simulink library "Ground_Source_Heat_Exchanger"  (R2018b)
settings: Solver=ode45  StartTime=0.0  StopTime=10.0  RelTol=1e-3  EnableMultiTasking=on
undefined symbols (not defined in the file): Ad, Ad0, Ar, Au, Au0, Bd, Bd0, Br, Bu, Bu0, c1, c33, c4, Cd, Cdl, Cr, Cu, Dd, DiameterLastPiece, dl, Dr, Du, gfunction, L1, r_Trichter, Rechenradius, T_null, t_start, t_Trichter, Tdown_0, Tearth_anf, Temperature, Tup_0
settings Model: Creator=lena.frank  LastModifiedBy=drhf
settings DataIOCC: LimitDataPoints=on  SaveFormat=Array  SignalLoggingSaveFormat=ModelDataLogs
settings OptimizationCC: ExpressionDepthLimit=2147483647  LifeSpan=inf
settings DebuggingCC: UnderspecifiedInitializationDetection=Classic  MergeDetectMultiDrivingBlocksExec=none  SolverPrmCheckMsg=warning  FcnCallInpInsideContextMsg=warning  StateNameClashWarn=warning  SFUnexpectedBacktrackingDiag=warning  SFNoUnconditionalDefaultTransitionDiag=warning  SFExecutionAtInitializationDiag=none
settings HardwareCC: ProdBitPerPointer=32  ProdBitPerSizeT=32  ProdBitPerPtrDiffT=32  ProdLargestAtomicFloat=None  ProdIntDivRoundTo=Undefined  ProdEndianess=Unspecified  ProdWordSize=32  ProdHWDeviceType=32-bit Generic
settings ModelReferenceCC: PropagateSignalLabelsOutOfModel=off
settings SFSimCC: SimUseLocalCustomCode=off
settings RTWCC: RTWUseLocalCustomCode=off
settings CodeAppCC: StateflowObjectComments=on
settings GRTTargetCC: TargetLangStandard=C89/C90 (ANSI)  GeneratePreprocessorConditionals=Disable all  CombineOutputUpdateFcns=off  GRTInterface=on
settings ConfigComp: CovMetricSettings=dw  CovHtmlReporting=on  CovSaveCumulativeToWorkspaceVar=on  CovSaveSingleToWorkspaceVar=on  CovExternalEMLEnable=off

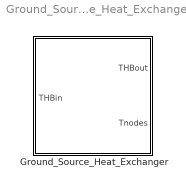
== system Ground_Source_Heat_Exchanger ==
  Ground_Source_Heat_Exchanger : Subsystem  mask(ground source heat exchanger){Jahresmitteltemp_C=10, TGrad=0.025, lambdaErde=2.5, cpErde=1000, rhoErde=2200, lambdaFill=0.81, cpFill=3040, rhoFill=1180, lambda_Sondenrohr=0.48, dTdesign=5, Sondenlaenge=100, B_sondenabstand=10, Sondendurchmesser=0.026+2*0.003, Bohrdurchmesser=0.12, Bu_param=0.06, Wanddicke_Sondenrohr=0.003, SondenFall=5x10 probes B/H = 0.1, DimVert=5, DimRad=10, Gitterfaktor=2.5, LastYear=1, show=off}
      mask prompts: Jahresmitteltemp_C "Average annual outdoor temperature  in °C"; TGrad "Temperature gradient in K/m, typical 0.025..0.04"; lambdaErde "Thermal conductivity ground in W/m/K"; cpErde "Heat capacity of the ground in J/kg/K"; rhoErde "Denstiy of the ground in kg/m³"; lambdaFill "Thermal conductivity filling in W/m/K"; cpFill "Heat capacity of the filling in J/kg/K"; rhoFill "Denstiy of the filling in kg/m³"; lambda_Sondenrohr "Thermal conductivity of pipe material  in W/m/K"; dTdesign "Design temperature difference inlet-outlet in K"; Sondenlaenge "H: Length of earth probe in m"; B_sondenabstand "B: Probe distance in m (= calculation diameter for single probe)"; Sondendurchmesser "Diameter of tube in m"; Bohrdurchmesser "Diameter of drilled hole in m"; Bu_param "Shank spacing in m (must be < borehole diameter)"; Wanddicke_Sondenrohr "Thickness of pipe wall in m"; SondenFall "Field geometry"; DimVert "No. of vertical nodes (typical 5, minimum 2)"; DimRad "No. of horizontal (radial) nodes (typical 10, minimum 3)"; Gitterfaktor "grid factor (typical 2.5, must be > 1)"; LastYear "Year of ground temperature pre-calculation (steady state = 50)"; show "Display start conditions"
      mask help: The CARNOT EWS model is a transient model for dynamic simulation of borehole heat exchangers or so-called vertical ground heat exchangers. The model is based on the equations described by [Huber] and has been implemented using the state space model of Matlab/Simulink [Bianchi]. See <Help> for literature.
      mask init:
      | startfall = 2;
      | DimAxi = max(DimVert*2,4);
      | DimRad = max(DimRad,3);
      | 
      | [Ad,Bd,Cd,Dd, Au,Bu,Cu,Du, Ad0,Bd0, Au0,Bu0, ...
      |     Ar,Br,Cr,Dr, Cdl, c1, c3, c31, c33, c4, c41, c5, c6, ...
      |     L1, L2, L10, L20, dl, Rechenradius, np, ...
      |     Tearth_anf, T_null, teta_fluid_ini, Tdown_0, Tup_0, ...
      |     Ts_Trichter, t_Trichter, r_Trichter, gfunction, t_start ...
      |     ] = ...
      |     CarnotCallbacks_EWS(startfall, LastYear, dTdesign, ...
      |     SondenFall, B_sondenabstand, Sondenlaenge, Sondendurchmesser, ...
      |     Bohrdurchmesser, Bu_param, Wanddicke_Sondenrohr, ...
      |     Jahresmitteltemp_C, TGrad, ...
      |     lambdaErde, rhoErde, cpErde, ...
      |     lambdaFill, cpFill, rhoFill, lambda_Sondenrohr, ...
      |     DimAxi, DimRad, Gitterfaktor, show);
      mask Help: web(fullfile(path_carnot('help'),'Ground_Source_Heat_Exchanger.html'),'-helpbrowser')
      mask TypeOptions SondenFall: 1 probe | 2 probes B/H = 0.1 | 2 probes B/H = 0.05 | 3x6 probes B/H = 0.1 | 5x10 probes B/H = 0.1
      mask DialogControl ParameterTabVar0 Prompt: Thermal
      mask DialogControl ParameterTabVar01 Prompt: Geometry
      mask DialogControl ParameterTabVar012 Prompt: Calculation
      mask Display:
      | plot(0,10,100,90,[70,30],[80,80], ...
      |     [35,35,43,43,47,52,57,57,66,66,60,60,54,46,40,40,35], ...
      |     [84,87,87,20,13,13,21,87,87,84,84,20,10,10,20,84,84])

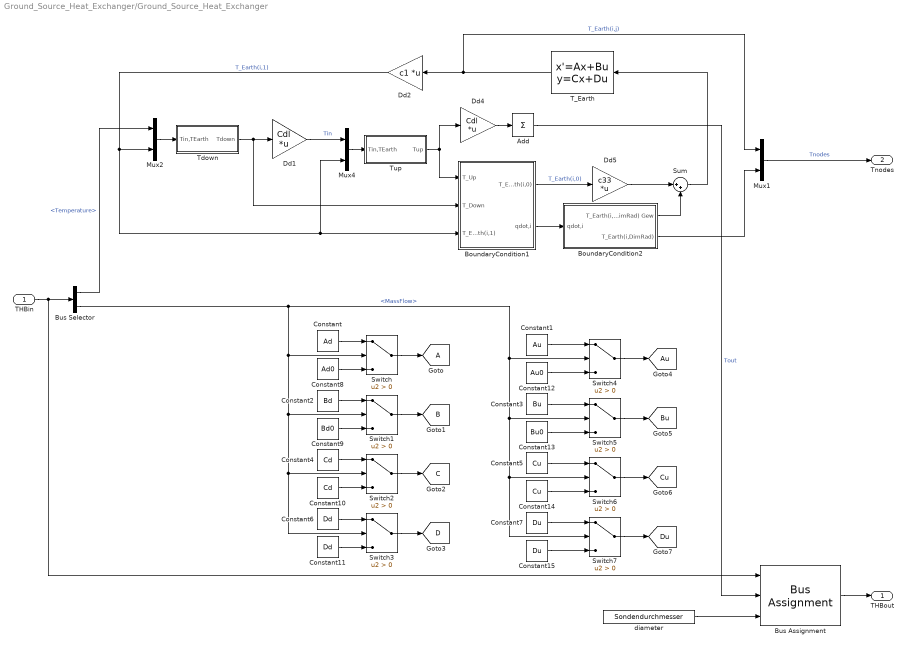
== system Ground_Source_Heat_Exchanger/Ground_Source_Heat_Exchanger ==
  THBin : Inport
  Add : Sum  Inputs=1
  BoundaryCondition1 : Subsystem
  BoundaryCondition2 : Subsystem
  Bus Assignment : BusAssignment  AssignedSignals=Temperature,DiameterLastPiece
  Bus Selector : BusSelector  OutputSignals=Temperature,MassFlow
  Constant : Constant  Value=Ad
  Constant1 : Constant  Value=Au
  Constant10 : Constant  Value=Cd
  Constant11 : Constant  Value=Dd
  Constant12 : Constant  Value=Au0
  Constant13 : Constant  Value=Bu0
  Constant14 : Constant  Value=Cu
  Constant15 : Constant  Value=Du
  Constant2 : Constant  Value=Bd
  Constant3 : Constant  Value=Bu
  Constant4 : Constant  Value=Cd
  Constant5 : Constant  Value=Cu
  Constant6 : Constant  Value=Dd
  Constant7 : Constant  Value=Du
  Constant8 : Constant  Value=Ad0
  Constant9 : Constant  Value=Bd0
  Dd1 : Gain  Gain=Cdl  Multiplication=Matrix(K*u)  SaturateOnIntegerOverflow=on  OutDataTypeStr=Inherit: Same as input  ParamDataTypeStr=Inherit: Same as input
  Dd2 : Gain  Gain=c1  Multiplication=Matrix(K*u)  SaturateOnIntegerOverflow=on  OutDataTypeStr=Inherit: Same as input  ParamDataTypeStr=Inherit: Same as input
  Dd4 : Gain  Gain=Cdl  Multiplication=Matrix(K*u)  SaturateOnIntegerOverflow=on  OutDataTypeStr=Inherit: Same as input  ParamDataTypeStr=Inherit: Same as input
  Dd5 : Gain  Gain=c33  Multiplication=Matrix(K*u)  SaturateOnIntegerOverflow=on  OutDataTypeStr=Inherit: Same as input  ParamDataTypeStr=Inherit: Same as input
  Mux1 : Mux  Inputs=2
  Mux2 : Mux  Inputs=2
  Mux4 : Mux  Inputs=2
  Sum : Sum  Inputs=|++  SaturateOnIntegerOverflow=on  InputSameDT=on  OutDataTypeStr=Inherit: Same as first input
  Switch{,1..7} (8 alike) : Switch  Criteria=u2 > Threshold
  T_Earth : StateSpace  A=Ar  B=Br  C=Cr  D=Dr  InitialCondition=Tearth_anf(:)
  Tdown : Subsystem
  Tup : Subsystem
  diameter : Constant  Value=Sondendurchmesser
  THBout : Outport
  Tnodes : Outport  Port=2
  tag scope: A=global, Au=global, B=global, Bu=global, C=global, Cu=global, D=global, Du=global
  wires:
  Bus Selector/1 -> Mux2/1  "<Temperature>"
  Bus Selector/2 -> Switch4/2, Switch5/2, Switch7/2, Switch6/2, Switch/2, Switch1/2, Switch3/2, Switch2/2  "<MassFlow>"
  Constant12/1 -> Switch4/3
  Constant13/1 -> Switch5/3
  Constant14/1 -> Switch6/3
  Constant15/1 -> Switch7/3
  Switch4/1 -> [Au]
  Switch5/1 -> [Bu]
  Switch6/1 -> [Cu]
  Switch7/1 -> [Du]
  Constant7/1 -> Switch7/1
  Constant5/1 -> Switch6/1
  Constant3/1 -> Switch5/1
  Constant1/1 -> Switch4/1
  Constant6/1 -> Switch3/1
  Constant11/1 -> Switch3/3
  Constant10/1 -> Switch2/3
  Switch3/1 -> [D]
  Constant4/1 -> Switch2/1
  Switch2/1 -> [C]
  Constant9/1 -> Switch1/3
  Constant2/1 -> Switch1/1
  Constant/1 -> Switch/1
  Switch1/1 -> [B]
  Constant8/1 -> Switch/3
  Switch/1 -> [A]
  Tdown/1(Tdown) -> Dd1/1, BoundaryCondition1/2(T_Down)
  Mux2/1 -> Tdown/1(Tin,TEarth)
  Mux4/1 -> Tup/1(Tin,TEarth)
  Dd1/1 -> Mux4/1  "Tin"
  T_Earth/1 -> Dd2/1, Mux1/1  "T_Earth(i,j)"
  Tup/1(Tup) -> Dd4/1, BoundaryCondition1/1(T_Up)
  Dd5/1 -> Sum/1
  BoundaryCondition2/1(T_Earth(i,DimRad) Gew) -> Sum/2
  Sum/1 -> T_Earth/1
  BoundaryCondition1/1(T_Earth(i,0)) -> Dd5/1  "T_Earth(i,0)"
  Dd2/1 -> Mux4/2, BoundaryCondition1/3(T_Earth(i,1)), Mux2/2  "T_Earth(i,1)"
  BoundaryCondition2/2(T_Earth(i,DimRad)) -> Mux1/2
  THBin/1 -> Bus Selector/1, Bus Assignment/1
  diameter/1 -> Bus Assignment/3
  Bus Assignment/1 -> THBout/1
  Dd4/1 -> Add/1
  Add/1 -> Bus Assignment/2  "Tout"
  Mux1/1 -> Tnodes/1  "Tnodes"
  BoundaryCondition1/2(qdot,i) -> BoundaryCondition2/1(qdot,i)

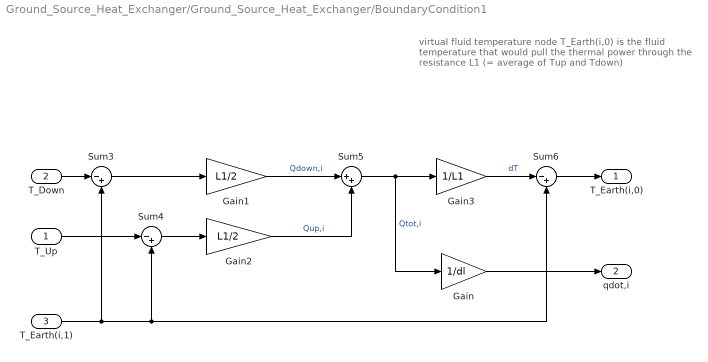
== system Ground_Source_Heat_Exchanger/Ground_Source_Heat_Exchanger/BoundaryCondition1 ==
  note: virtual fluid temperature node T_Earth(i,0) is the
      | fluid temperature that would pull the thermal
      | power through the resistance L1 (= average of
      | Tup and Tdown)
  T_Up : Inport
  T_Down : Inport  Port=2
  T_Earth(i,1) : Inport  Port=3
  Gain : Gain  Gain=1/dl
  Gain1 : Gain  Gain=L1/2  SaturateOnIntegerOverflow=on  OutDataTypeStr=Inherit: Same as input  ParamDataTypeStr=Inherit: Same as input
  Gain2 : Gain  Gain=L1/2  SaturateOnIntegerOverflow=on  OutDataTypeStr=Inherit: Same as input  ParamDataTypeStr=Inherit: Same as input
  Gain3 : Gain  Gain=1/L1  SaturateOnIntegerOverflow=on  OutDataTypeStr=Inherit: Same as input  ParamDataTypeStr=Inherit: Same as input
  Sum3 : Sum  Inputs=|-+  SaturateOnIntegerOverflow=on  InputSameDT=on  OutDataTypeStr=Inherit: Same as first input
  Sum4 : Sum  Inputs=|-+  SaturateOnIntegerOverflow=on  InputSameDT=on  OutDataTypeStr=Inherit: Same as first input
  Sum5 : Sum  Inputs=|++  SaturateOnIntegerOverflow=on  InputSameDT=on  OutDataTypeStr=Inherit: Same as first input
  Sum6 : Sum  Inputs=|-+  SaturateOnIntegerOverflow=on  InputSameDT=on  OutDataTypeStr=Inherit: Same as first input
  T_Earth(i,0) : Outport
  qdot,i : Outport  Port=2
  wires:
  Sum3/1 -> Gain1/1
  Sum4/1 -> Gain2/1
  Gain1/1 -> Sum5/1  "Qdown,i"
  Gain2/1 -> Sum5/2  "Qup,i"
  Sum5/1 -> Gain/1, Gain3/1  "Qtot,i"
  Gain3/1 -> Sum6/1  "dT"
  T_Down/1 -> Sum3/1
  T_Up/1 -> Sum4/1
  T_Earth(i,1)/1 -> Sum3/2, Sum6/2, Sum4/2
  Sum6/1 -> T_Earth(i,0)/1
  Gain/1 -> qdot,i/1

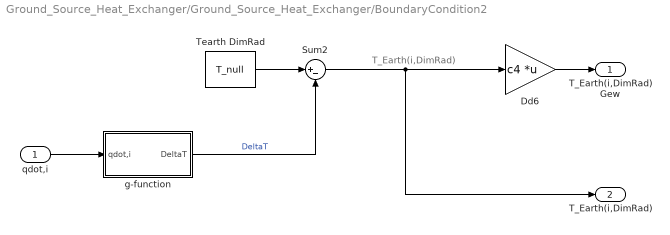
== system Ground_Source_Heat_Exchanger/Ground_Source_Heat_Exchanger/BoundaryCondition2 ==
  note: T_Earth(i,DimRad)
  qdot,i : Inport
  Dd6 : Gain  Gain=c4  Multiplication=Matrix(K*u)  SaturateOnIntegerOverflow=on  OutDataTypeStr=Inherit: Same as input  ParamDataTypeStr=Inherit: Same as input
  Sum2 : Sum  Inputs=|+-  SaturateOnIntegerOverflow=on  InputSameDT=on  OutDataTypeStr=Inherit: Same as first input
  Tearth DimRad : Constant  Value=T_null  VectorParams1D=off
  g-function : Subsystem
  T_Earth(i,DimRad) Gew : Outport
  T_Earth(i,DimRad) : Outport  Port=2
  wires:
  g-function/1(DeltaT) -> Sum2/2  "DeltaT"
  Dd6/1 -> T_Earth(i,DimRad) Gew/1
  qdot,i/1 -> g-function/1(qdot,i)
  Tearth DimRad/1 -> Sum2/1
  Sum2/1 -> T_Earth(i,DimRad)/1, Dd6/1

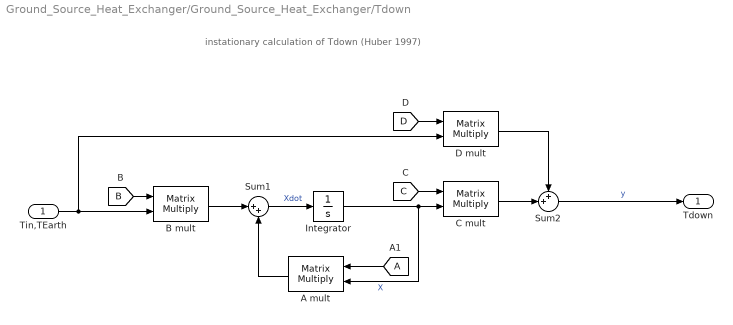
== system Ground_Source_Heat_Exchanger/Ground_Source_Heat_Exchanger/Tdown ==
  note: instationary calculation of Tdown (Huber 1997)
  Tin,TEarth : Inport
  A mult : Product  Multiplication=Matrix(*)  RndMeth=Zero
  B mult : Product  Multiplication=Matrix(*)  RndMeth=Zero
  C mult : Product  Multiplication=Matrix(*)  RndMeth=Zero
  D mult : Product  Multiplication=Matrix(*)  RndMeth=Zero
  Integrator : Integrator  InitialCondition=Tdown_0
  Sum1 : Sum  Inputs=|++
  Sum2 : Sum  Inputs=++|
  Tdown : Outport
  wires:
  [D] -> D mult/1
  [C] -> C mult/1
  [A] -> A mult/1
  [B] -> B mult/1
  A mult/1 -> Sum1/2
  Integrator/1 -> C mult/2, A mult/2  "X"
  Sum1/1 -> Integrator/1  "Xdot"
  B mult/1 -> Sum1/1
  C mult/1 -> Sum2/2
  D mult/1 -> Sum2/1
  Tin,TEarth/1 -> D mult/2, B mult/2
  Sum2/1 -> Tdown/1  "y"

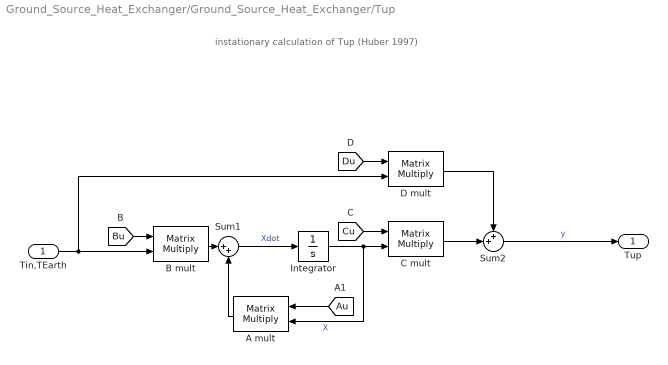
== system Ground_Source_Heat_Exchanger/Ground_Source_Heat_Exchanger/Tup ==
  note: instationary calculation of Tup (Huber 1997)
  Tin,TEarth : Inport
  A mult : Product  Multiplication=Matrix(*)  RndMeth=Zero
  B mult : Product  Multiplication=Matrix(*)  RndMeth=Zero
  C mult : Product  Multiplication=Matrix(*)  RndMeth=Zero
  D mult : Product  Multiplication=Matrix(*)  RndMeth=Zero
  Integrator : Integrator  InitialCondition=Tup_0
  Sum1 : Sum  Inputs=|++
  Sum2 : Sum  Inputs=++|
  Tup : Outport
  wires:
  [Du] -> D mult/1
  [Cu] -> C mult/1
  [Au] -> A mult/1
  [Bu] -> B mult/1
  A mult/1 -> Sum1/2
  Integrator/1 -> C mult/2, A mult/2  "X"
  Sum1/1 -> Integrator/1  "Xdot"
  B mult/1 -> Sum1/1
  C mult/1 -> Sum2/2
  D mult/1 -> Sum2/1
  Tin,TEarth/1 -> D mult/2, B mult/2
  Sum2/1 -> Tup/1  "y"

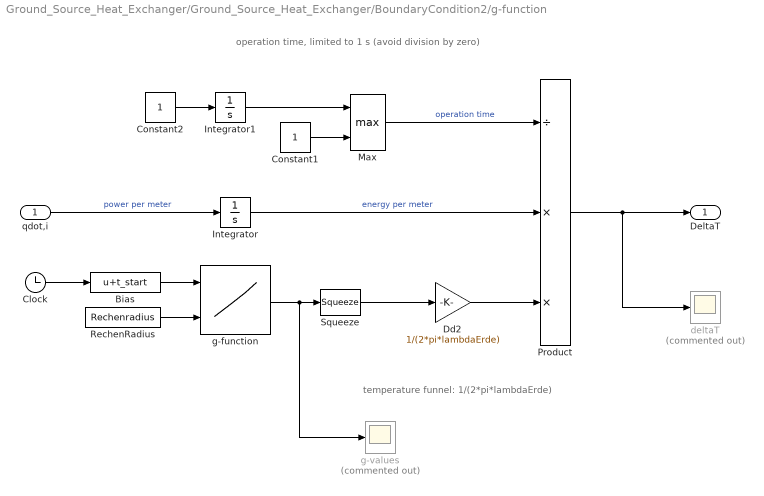
== system Ground_Source_Heat_Exchanger/Ground_Source_Heat_Exchanger/BoundaryCondition2/g-function ==
  note: operation time, limited to 1 s (avoid division by zero)
  note: temperature funnel: 1/(2*pi*lambdaErde)
  qdot,i : Inport
  Bias : Bias  Bias=t_start
  Clock : Clock
  Constant1 : Constant
  Constant2 : Constant
  Dd2 : Gain  Gain=1/(2*pi*lambdaErde)  SaturateOnIntegerOverflow=on  OutDataTypeStr=Inherit: Same as input  ParamDataTypeStr=Inherit: Same as input
  Integrator : Integrator
  Integrator1 : Integrator  LowerSaturationLimit=1
  Max : MinMax  Function=max  Inputs=2
  Product : Product  Inputs=/**  SaturateOnIntegerOverflow=on  RndMeth=Zero  InputSameDT=on  OutDataTypeStr=Inherit: Same as first input
  RechenRadius : Constant  Value=Rechenradius  VectorParams1D=off
  Squeeze : Squeeze
  deltaT : Scope  Commented=on
  g-function : Lookup_n-D  BreakpointsForDimension1=t_Trichter  BreakpointsForDimension2=r_Trichter  BeginIndexSearchUsingPreviousIndexResult=on  Table=gfunction  InternalRulePriority=Speed  RndMeth=Simplest  InputSameDT=on
  g-values : Scope  Commented=on
  DeltaT : Outport
  wires:
  RechenRadius/1 -> g-function/2
  Dd2/1 -> Product/3
  Product/1 -> deltaT/1, DeltaT/1
  g-function/1 -> g-values/1, Squeeze/1
  qdot,i/1 -> Integrator/1  "power per meter"
  Squeeze/1 -> Dd2/1
  Integrator/1 -> Product/2  "energy per meter"
  Integrator1/1 -> Max/1
  Constant1/1 -> Max/2
  Max/1 -> Product/1  "operation time"
  Constant2/1 -> Integrator1/1
  Clock/1 -> Bias/1
  Bias/1 -> g-function/1
